simulink model "ej4simulink"  (R2024b)
settings: Solver=ode4  StartTime=0.0  StopTime=10  FixedStep=0.0001  RelTol=1e-3
values from neighbouring files (symbols this model uses):
  ue = 1/2    (= 0.5)    [modelizacion150824.m]    (also in punto4.m)
  x_e = [3; 2; 1; 1]    [modelizacion150824.m]
  ye = 1    [punto4.m]
libraries: cstblocks x1
settings Model: Creator=aghersin  LastModifiedBy=maxirodriguez
settings SolverCC: AlgebraicLoopSolver=TrustRegion
settings DataIOCC: ReturnWorkspaceOutputs=off
settings OptimizationCC: LifeSpan=inf
settings DebuggingCC: UnconnectedInputMsg=warning  UnconnectedOutputMsg=warning  UnconnectedLineMsg=warning  SFExecutionAtInitializationDiag=none  ArithmeticOperatorsInVariantConditions=warning
settings ModelReferenceCC: EnableRefExpFcnMdlSchedulingChecks=on
settings SFSimCC: SimUseLocalCustomCode=off  CustomCodeUndefinedFunction=UseInterfaceOnly
settings RTWCC: RTWUseLocalCustomCode=off  GPUComputeCapability=3.5
settings CodeAppCC: StateflowObjectComments=on

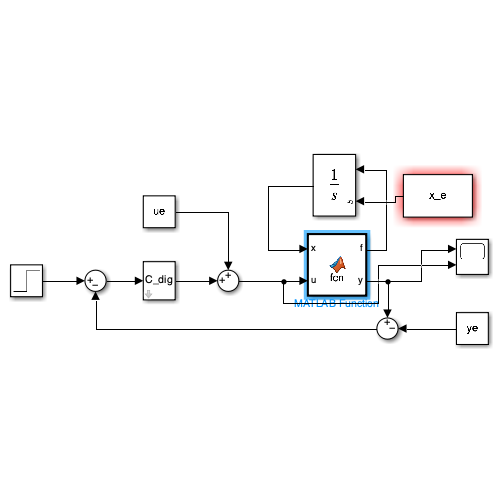
[thumbnail: Simulink's stored preview of the top-level diagram]
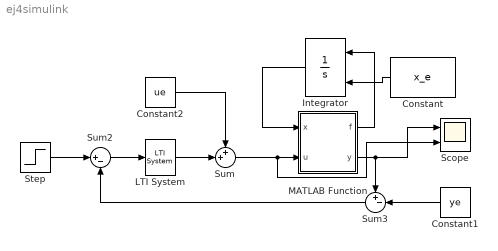
== system ej4simulink ==
  Constant : Constant  Value=x_e
  Constant1 : Constant  Value=ye
  Constant2 : Constant  Value=ue
  Integrator : Integrator  InitialConditionSource=external
  LTI System : cstblocks/LTI System  sys=C_dig  IC=[]  PadeOrder=0
  MATLAB Function : MATLAB Function  TreatAsAtomicUnit=on
  Scope : Scope  NumInputPorts=2
  Step : Step  Time=0  After=0.1  SampleTime=0
  Sum : Sum  Inputs=++|
  Sum2 : Sum  Inputs=|+-
  Sum3 : Sum  Inputs=+-|
  wires:
  Integrator/1 -> MATLAB Function/1(x)
  MATLAB Function/1(f) -> Integrator/1
  Constant/1 -> Integrator/2
  MATLAB Function/2(y) -> Sum3/1, Scope/1
  Constant1/1 -> Sum3/2
  Constant2/1 -> Sum/1
  Sum2/1 -> LTI System/1
  Step/1 -> Sum2/1
  Sum3/1 -> Sum2/2
  LTI System/1 -> Sum/2
  Sum/1 -> Scope/2, MATLAB Function/2(u)

== matlab function ej4simulink/MATLAB Function ==
  data: x input; u input; f output; y output
function [f,y] = fcn(x,u)

f1 = (x(3)-sqrt((x(1)-x(2))))/(x(1)^2);

f2 = (sqrt((x(1)-x(2)))-sqrt((x(2))))/(x(2)^2);

f3 = x(4);
f4 = x(5);
f5 = x(6);

f6 = (u - (1/2)*x(6) - (3/2)*x(5) - 2*x(4) - x(3)) * 16;


f = [f1;f2;f3;f4;f5;f6];

%defino la salida
y = x(2);
